simulink model "XYZCartesianRobot3DPrinting"  (R2024a)
settings: Solver=daessc  StartTime=0.0  StopTime=30  RelTol=1e-3  AbsTol=1e-3
PostLoadFcn:
  | run('XYZGantryRobotParameters.m')
  | run('LoadGantryRobot');
undefined symbols (not defined in the file): Controller, Floor, PrintBed, PrintHead, Trajectory, X, Y, Z
libraries: fl_lib x22, slpidlib x22, nesl_utility x15, sm_lib x10, sdl_lib x6, simulink x6, ee_lib x3
(part 1 of 3)
settings Model: Creator=abirdas  LastModifiedBy=abirdas
settings SolverCC: AutoScaleAbsTol=off
settings DataIOCC: SignalLoggingName=logsoutCartesianRobot3DPrinting
settings SimscapeCC: SimscapeLogType=all  SimscapeLogDataHistory=10000000

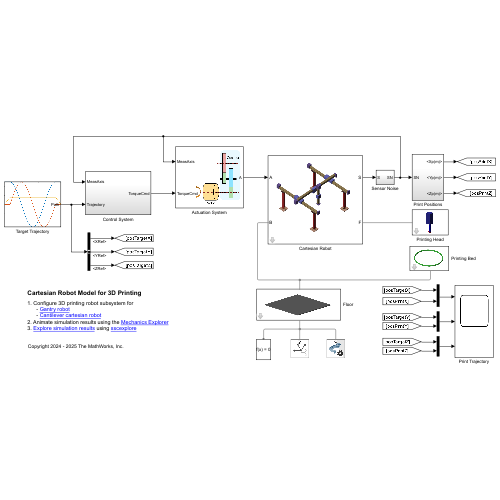
[thumbnail: Simulink's stored preview of the top-level diagram]
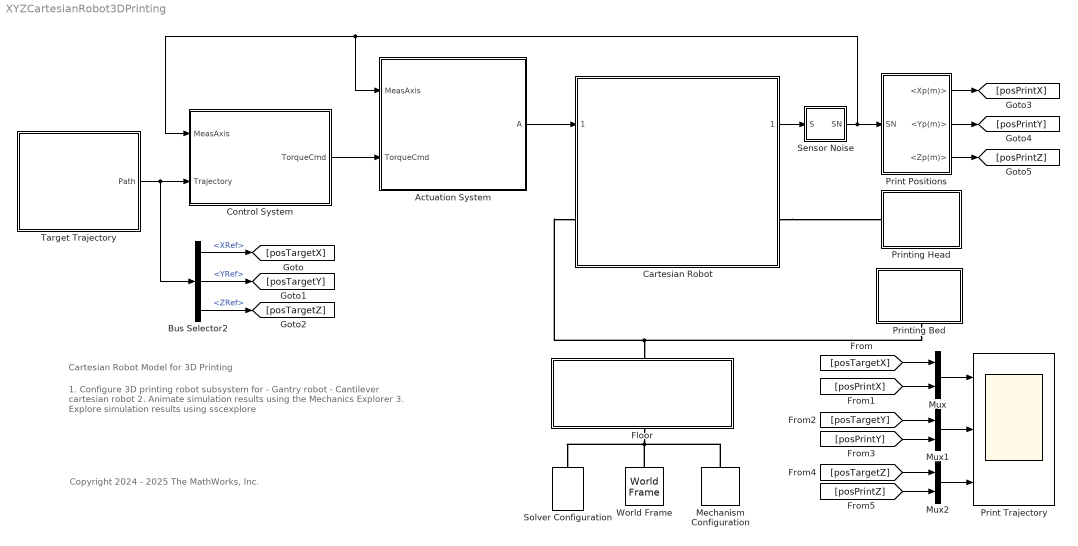
== system XYZCartesianRobot3DPrinting ==
  note: 1. Configure 3D printing robot subsystem for
      | - Gantry robot
      | - Cantilever cartesian robot
      | 2. Animate simulation results using the Mechanics Explorer
      | 3. Explore simulation results using sscexplore
  note: Cartesian Robot Model for 3D Printing
  note: Copyright 2024 - 2025 The MathWorks, Inc.
  Actuation System : Subsystem
      mask Display: image('ElectricalActuationSystem.png');
  Bus Selector2 : BusSelector  OutputSignals=XRef,YRef,ZRef
  Cartesian Robot : Subsystem  ReferencedSubsystem=GantryRobotSubsystem  DOF=3DOF  configAxis=XYZ  heightColumn=CartesianRobot.BaseFrame.heightColumn  widthColumn=CartesianRobot.BaseFrame.widthColumn  positionColumn1=CartesianRobot.BaseFrame.positionColumn1  positionColumn2=CartesianRobot.BaseFrame.positionColumn2  positionColumn3=CartesianRobot.BaseFrame.positionColumn3  positionColumn4=CartesianRobot.BaseFrame.positionColumn4  systemGuideX=Rail-block  strokeXMax=CartesianRobot.XAxis.strokeMax  widthGuideX=CartesianRobot.XAxis.widthRail  diaScrewX=0.05  widthXMount=0.3  typeInertiaGuideX=Calculate from Geometry  densityGuideX=CartesianRobot.XAxis.densityRail  massGuideX=0  COMGuideX=0  MOIGuideX=0  POIGuideX=0  typeInertiaCarriageX=Calculate from Geometry  densityCarriageX=CartesianRobot.XAxis.densityBlock  massCarriageX=0  COMCarriageX=0  MOICarriageX=0  POICarriageX=0  colorGuideX=[0.7 0.6 0.4]  colorCarriageX=[0.5 0.5 0.9]  systemGuideY=Rail-block  strokeYMax=CartesianRobot.YAxis.strokeMax  widthGuideY=CartesianRobot.YAxis.widthRail  diaScrewY=0.05  widthYMount=0.15  typeInertiaGuideY=Calculate from Geometry  densityGuideY=CartesianRobot.YAxis.densityRail  massGuideY=0  COMGuideY=0  MOIGuideY=0  POIGuideY=0  typeInertiaCarriageY=Calculate from Geometry  densityCarriageY=CartesianRobot.YAxis.densityBlock  massCarriageY=0  COMCarriageY=0  MOICarriageY=0  POICarriageY=0  colorGuideY=[0.7 0.6 0.4]  colorCarriageY=[0.5 0.5 0.9]  systemGuideZ=Rail-block  strokeZMax=CartesianRobot.ZAxis.strokeMax  widthGuideZ=CartesianRobot.ZAxis.widthRail  diaScrewZ=0.05  shiftZAxisDown=CartesianRobot.ZAxis.shiftZAxisDown  widthZMount=0.15  typeInertiaGuideZ=Calculate from Geometry  densityGuideZ=CartesianRobot.ZAxis.densityRail  massGuideZ=0  COMGuideZ=0  MOIGuideZ=0  POIGuideZ=0  typeInertiaCarriageZ=Calculate from Geometry  densityCarriageZ=CartesianRobot.ZAxis.densityBlock  massCarriageZ=0  COMCarriageZ=0  MOICarriageZ=0  POICarriageZ=0  colorGuideZ=[0.7 0.6 0.4]  colorCarriageZ=[0.5 0.5 0.9]
  Control System : Subsystem
  Floor : Subsystem  mask{floorDims=Floor.dimensions, floorPos=Floor.position}
      mask prompts: floorDims "Floor dimensions (m)"; floorPos "Floor position (m)"
      settings: PortSchema="{\"entries\":[{\"content\":{\"sides\":[{\"content\":{},\"type\":\"ConnectorPlacement.EquallySpacedRectSide\",\"uuid\":\"5b485af5-4f05-4248-a7f3-08377bf9cff2\"},{\"content\":{\"side\":\"RIGHT\"},\"type\":\"ConnectorPlacement.EquallySpacedRectSide\",\"uuid\":\"824380b3-967b-4422-aed9-09760effc9b4\"},{\"content\":{\"connectorIds\":[\"LConn1\"],\"side\":\"TOP\"},\"type\":\"ConnectorPlacement.EquallySpacedRectSide\",\"uuid\":\"4c7d634e-a270-49ee-a9b6-ce866eb97663\"},{\"content\":{\"connectorIds\":[\"RConn1\"],\"side\":\"BOTTOM\"},\"type\":\"ConnectorPlacement.EquallySpacedRectSide\",\"uuid\":\"d939dd98-fa2d-4b24-975e-597412481fcf\"}]},\"type\":\"ConnectorPlacement.EquallySpacedConnector\",\"uuid\":\"704e5fa1-0bef-4b5b-a1a4-570354550c26\"}],\"packageUris\":[\"http://schema.mathworks.com/mf0/Connector/R2020b\"],\"version\":\"1.0\"}"
      mask Display: image('Floor.png');
  Mechanism Configuration : sm_lib/Utilities/Mechanism Configuration  UniformGravity=Constant  GravityVector=[0 0 -9.80665]  GravityVectorUnits=m/s^2  LinearizationDelta=0.001  JointModeTransitionNonlinearIterations=2
  Mux : Mux  Inputs=2
  Mux1 : Mux  Inputs=2
  Mux2 : Mux  Inputs=2
  Print Positions : Subsystem
  Print Trajectory : Scope  NumInputPorts=3
  Printing Bed : Subsystem  mask{bedOffset=PrintBed.offsetFloor, bedRadius=PrintBed.radiusCircle, bedHeight=PrintBed.height, penThk=PrintHead.diaNozzleExit}
      mask prompts: bedOffset "Printing bed offset from floor (m)"; bedRadius "Printing bed radius (m)"; bedHeight "Printing bed height (m)"; penThk "Printing pen thickness (m)"
      mask init:
      | % Vertices of circular printing bed
      | v1 = [bedRadius + 0.5*penThk, 0];
      | v2 = [bedRadius + 0.5*penThk, bedHeight];
      | v3 = [bedRadius - 0.5*penThk, bedHeight];
      | v4 = [bedRadius - 0.5*penThk, 0];
      | sectionCircPrint = [v1; v2; v3; v4];
      settings: PortSchema="{\"entries\":[{\"content\":{\"sides\":[{\"content\":{},\"type\":\"ConnectorPlacement.EquallySpacedRectSide\",\"uuid\":\"5b485af5-4f05-4248-a7f3-08377bf9cff2\"},{\"content\":{\"side\":\"RIGHT\"},\"type\":\"ConnectorPlacement.EquallySpacedRectSide\",\"uuid\":\"824380b3-967b-4422-aed9-09760effc9b4\"},{\"content\":{\"side\":\"TOP\"},\"type\":\"ConnectorPlacement.EquallySpacedRectSide\",\"uuid\":\"4c7d634e-a270-49ee-a9b6-ce866eb97663\"},{\"content\":{\"connectorIds\":[\"RConn1\"],\"side\":\"BOTTOM\"},\"type\":\"ConnectorPlacement.EquallySpacedRectSide\",\"uuid\":\"d939dd98-fa2d-4b24-975e-597412481fcf\"}]},\"type\":\"ConnectorPlacement.EquallySpacedConnector\",\"uuid\":\"704e5fa1-0bef-4b5b-a1a4-570354550c26\"}],\"packageUris\":[\"http://schema.mathworks.com/mf0/Connector/R2020b\"],\"version\":\"1.0\"}"
      mask Display: image('AnnularPrintingBed.png');
  Printing Head : Subsystem  mask{dNozzle=PrintHead.diaNozzleExit}
      mask prompts: dNozzle "Nozzle exit diameter (m)"
      mask Display: image('PrintHead.png');
  Sensor Noise : Subsystem
  Solver Configuration : nesl_utility/Solver Configuration  PhysicalDomain=network_engine_domain  SubClassName=solver  LeftPortType=input  RightPortType=generic  Tones=[]  Harmonics=[]  SimulateNoise=off  Profile=off  UseLocalSampling=off  EnableSwitchedLinearOptims=on  FrequencyDomain=off  UseCCode=off  RelTol=0.001  AbsTol=0.001  MinStep=1e-09  ToWorkspace=off  RevertToSquareIcSolve=off  NumHomotopyIterations=100  PhasorMode=off  PhasorModeNumHarmonics=1  ConsistencySolver=NEWTON_XTOL_AFTER_FTOL  IndexReductionMethod=DerivativeReplacement  DoDC=off  ResidualTolerance=1e-09  ConsistencyTolSource=GLOBAL  ConsistencyAbsTol=0.001  ConsistencyRelTol=0.001  ConsistencyTolFactor=0.001  UseLocalSolver=off  LocalSolverChoice=NE_BACKWARD_EULER_ADVANCER  ResolveIndetEquations=on  FunctionEvalNumThread=1  LocalSolverSampleTime=0.001  DoFixedCost=off  MaxNonlinIter=3  MaxModeIter=2  ComputeImpulses=off  ImpulseIterations=2  LinearAlgebra=auto  LinearAlgebraNumThread=0  EquationFormulation=NE_TIME_EF  DelaysMemoryBudget=1024  AutomaticFiltering=on  FilteringTimeConstant=0.001  PartitionStorageMethod=AS_NEEDED  PartitionMemoryBudget=1024  PartitionMethod=ROBUST  MultibodyUseLocalSolver=off  MultibodyLocalSolverChoice=ODE1  MultibodyLocalSolverSampleTime=0.001
  Target Trajectory : Subsystem
      mask Display: image('MotionInputs.png');
  World Frame : sm_lib/Frames and Transforms/World Frame
  wires:
  Control System/1(TorqueCmd) -> Actuation System/2(TorqueCmd)
  Actuation System/1(A) -> Cartesian Robot/1
  Target Trajectory/1(Path) -> Control System/2(Trajectory), Bus Selector2/1
  Bus Selector2/3 -> [posTargetZ]  "<ZRef>"
  Bus Selector2/1 -> [posTargetX]  "<XRef>"
  Bus Selector2/2 -> [posTargetY]  "<YRef>"
  [posTargetY] -> Mux1/1
  Mux1/1 -> Print Trajectory/2
  Mux/1 -> Print Trajectory/1
  [posPrintZ] -> Mux2/2
  [posTargetZ] -> Mux2/1
  Mux2/1 -> Print Trajectory/3
  [posPrintX] -> Mux/2
  [posPrintY] -> Mux1/2
  [posTargetX] -> Mux/1
  Cartesian Robot/1 -> Sensor Noise/1(S)
  Sensor Noise/1(SN) -> Actuation System/1(MeasAxis), Control System/1(MeasAxis), Print Positions/1(SN)
  Print Positions/1(<Xp(m)>) -> [posPrintX]
  Print Positions/2(<Yp(m)>) -> [posPrintY]
  Print Positions/3(<Zp(m)>) -> [posPrintZ]
  connections:
  World Frame/RConn1 -- Solver Configuration/RConn1 -- Mechanism Configuration/RConn1 -- Floor/RConn1
  Printing Bed/RConn1 -- Cartesian Robot/LConn1 -- Floor/LConn1
  Cartesian Robot/RConn1 -- Printing Head/LConn1

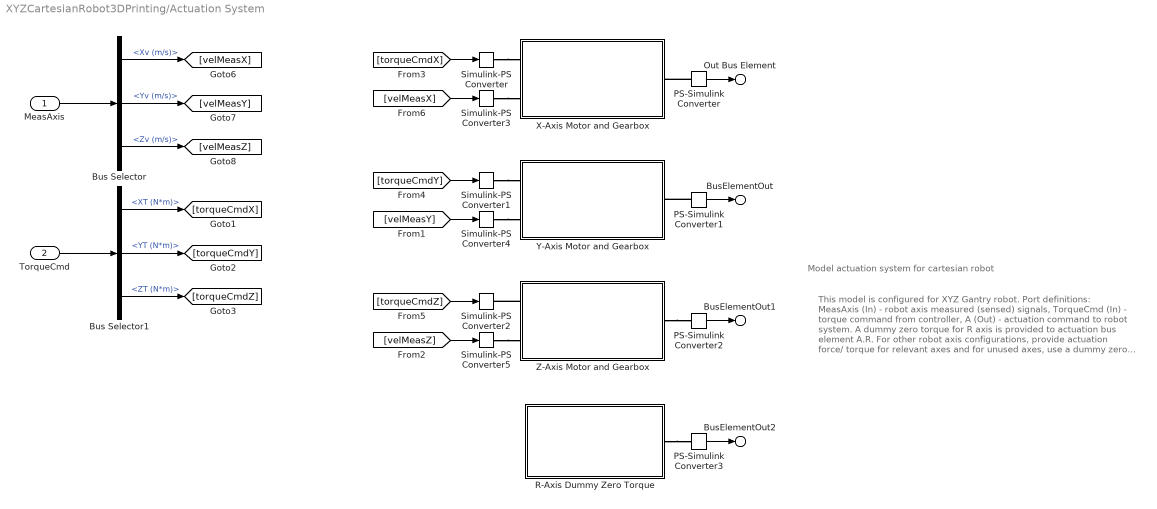
== system XYZCartesianRobot3DPrinting/Actuation System ==
  note: Model actuation system for cartesian robot
  note: This model is configured for XYZ Gantry robot.
      | Port definitions:
      | MeasAxis (In) - robot axis measured (sensed) signals,
      | TorqueCmd (In) - torque command from controller,
      | A (Out) - actuation command to robot system.
      |
      | A dummy zero torque for R axis is provided to actuation bus element A.R.
      | For other robot axis configurations, provide actuation force/ torque for relevant axes and for unused axes, use a dummy zero force/ torque.
  MeasAxis : Inport
  TorqueCmd : Inport  Port=2
  Bus Selector : BusSelector  OutputSignals=Xv (m/s),Yv (m/s),Zv (m/s)
  Bus Selector1 : BusSelector  OutputSignals=XT (N*m),YT (N*m),ZT (N*m)
  PS-Simulink Converter{,1..3} (4 alike) : nesl_utility/PS-Simulink Converter  PhysicalDomain=network_engine_domain  SubClassName=ps_output  LeftPortType=input  RightPortType=output  PseudoPeriodic=off  Frequencies=[]  VectorFormat=inherit  Unit=inherit  AffineConversion=off
  R-Axis Dummy Zero Torque : Subsystem
  Simulink-PS Converter : nesl_utility/Simulink-PS Converter  PhysicalDomain=network_engine_domain  SubClassName=ps_input  LeftPortType=input  RightPortType=output  PseudoPeriodic=off  Frequencies=[]  NoiseDistribution=none  NoiseParameters=[]  Unit=N*m  AffineConversion=off  FilteringAndDerivatives=provide  SimscapeFilterOrder=1  InputFilterTimeConstant=0.001  UdotUserProvided=0
  Simulink-PS Converter1 : nesl_utility/Simulink-PS Converter  PhysicalDomain=network_engine_domain  SubClassName=ps_input  LeftPortType=input  RightPortType=output  PseudoPeriodic=off  Frequencies=[]  NoiseDistribution=none  NoiseParameters=[]  Unit=N*m  AffineConversion=off  FilteringAndDerivatives=provide  SimscapeFilterOrder=1  InputFilterTimeConstant=0.001  UdotUserProvided=0
  Simulink-PS Converter2 : nesl_utility/Simulink-PS Converter  PhysicalDomain=network_engine_domain  SubClassName=ps_input  LeftPortType=input  RightPortType=output  PseudoPeriodic=off  Frequencies=[]  NoiseDistribution=none  NoiseParameters=[]  Unit=N*m  AffineConversion=off  FilteringAndDerivatives=provide  SimscapeFilterOrder=1  InputFilterTimeConstant=0.001  UdotUserProvided=0
  Simulink-PS Converter3 : nesl_utility/Simulink-PS Converter  PhysicalDomain=network_engine_domain  SubClassName=ps_input  LeftPortType=input  RightPortType=output  PseudoPeriodic=off  Frequencies=[]  NoiseDistribution=none  NoiseParameters=[]  Unit=m/s  AffineConversion=off  FilteringAndDerivatives=filter  SimscapeFilterOrder=1  InputFilterTimeConstant=0.001  UdotUserProvided=0
  Simulink-PS Converter4 : nesl_utility/Simulink-PS Converter  PhysicalDomain=network_engine_domain  SubClassName=ps_input  LeftPortType=input  RightPortType=output  PseudoPeriodic=off  Frequencies=[]  NoiseDistribution=none  NoiseParameters=[]  Unit=m/s  AffineConversion=off  FilteringAndDerivatives=filter  SimscapeFilterOrder=1  InputFilterTimeConstant=0.001  UdotUserProvided=0
  Simulink-PS Converter5 : nesl_utility/Simulink-PS Converter  PhysicalDomain=network_engine_domain  SubClassName=ps_input  LeftPortType=input  RightPortType=output  PseudoPeriodic=off  Frequencies=[]  NoiseDistribution=none  NoiseParameters=[]  Unit=m/s  AffineConversion=off  FilteringAndDerivatives=filter  SimscapeFilterOrder=1  InputFilterTimeConstant=0.001  UdotUserProvided=0
  X-Axis Motor and Gearbox : Subsystem
  Y-Axis Motor and Gearbox : Subsystem
  Z-Axis Motor and Gearbox : Subsystem
  Out Bus Element : Outport  PortName=A  Element=X
  BusElementOut : Outport  PortName=A  Element=Y
  BusElementOut1 : Outport  PortName=A  Element=Z
  BusElementOut2 : Outport  PortName=A  Element=R
  wires:
  MeasAxis/1 -> Bus Selector/1
  TorqueCmd/1 -> Bus Selector1/1
  Bus Selector1/1 -> [torqueCmdX]  "<XT (N*m)>"
  Bus Selector1/2 -> [torqueCmdY]  "<YT (N*m)>"
  Bus Selector1/3 -> [torqueCmdZ]  "<ZT (N*m)>"
  PS-Simulink Converter/1 -> Out Bus Element/1
  PS-Simulink Converter1/1 -> BusElementOut/1
  [velMeasX] -> Simulink-PS Converter3/1
  [velMeasY] -> Simulink-PS Converter4/1
  [velMeasZ] -> Simulink-PS Converter5/1
  [torqueCmdX] -> Simulink-PS Converter/1
  [torqueCmdY] -> Simulink-PS Converter1/1
  [torqueCmdZ] -> Simulink-PS Converter2/1
  PS-Simulink Converter3/1 -> BusElementOut2/1
  PS-Simulink Converter2/1 -> BusElementOut1/1
  Bus Selector/1 -> [velMeasX]  "<Xv (m/s)>"
  Bus Selector/2 -> [velMeasY]  "<Yv (m/s)>"
  Bus Selector/3 -> [velMeasZ]  "<Zv (m/s)>"
  connections:
  Z-Axis Motor and Gearbox/LConn1 -- Simulink-PS Converter2/RConn1
  Simulink-PS Converter/RConn1 -- X-Axis Motor and Gearbox/LConn1
  Simulink-PS Converter1/RConn1 -- Y-Axis Motor and Gearbox/LConn1
  PS-Simulink Converter/LConn1 -- X-Axis Motor and Gearbox/RConn1
  PS-Simulink Converter1/LConn1 -- Y-Axis Motor and Gearbox/RConn1
  Z-Axis Motor and Gearbox/RConn1 -- PS-Simulink Converter2/LConn1
  Simulink-PS Converter3/RConn1 -- X-Axis Motor and Gearbox/LConn2
  Simulink-PS Converter4/RConn1 -- Y-Axis Motor and Gearbox/LConn2
  Simulink-PS Converter5/RConn1 -- Z-Axis Motor and Gearbox/LConn2
  R-Axis Dummy Zero Torque/RConn1 -- PS-Simulink Converter3/LConn1

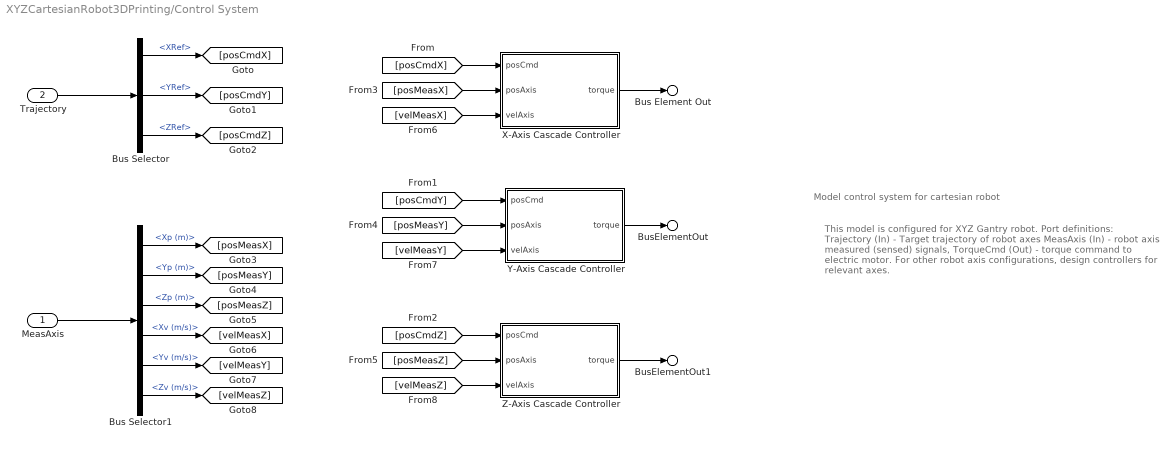
== system XYZCartesianRobot3DPrinting/Control System ==
  note: This model is configured for XYZ Gantry robot.
      | Port definitions:
      | Trajectory (In) - Target trajectory of robot axes
      | MeasAxis (In) - robot axis measured (sensed) signals,
      | TorqueCmd (Out) - torque command to electric motor.
      |
      | For other robot axis configurations, design controllers for relevant axes.
  note: Model control system for cartesian robot
  MeasAxis : Inport
  Trajectory : Inport  Port=2
  Bus Selector : BusSelector  OutputSignals=XRef,YRef,ZRef
  Bus Selector1 : BusSelector  OutputSignals=Xp (m),Yp (m),Zp (m),Xv (m/s),Yv (m/s),Zv (m/s)
  X-Axis Cascade Controller : Subsystem
  Y-Axis Cascade Controller : Subsystem
  Z-Axis Cascade Controller : Subsystem
  Bus Element Out : Outport  PortName=TorqueCmd  Element=XT (N*m)
  BusElementOut : Outport  PortName=TorqueCmd  Element=YT (N*m)
  BusElementOut1 : Outport  PortName=TorqueCmd  Element=ZT (N*m)
  wires:
  Trajectory/1 -> Bus Selector/1
  MeasAxis/1 -> Bus Selector1/1
  Bus Selector/1 -> [posCmdX]  "<XRef>"
  [posCmdX] -> X-Axis Cascade Controller/1(posCmd)
  Bus Selector/2 -> [posCmdY]  "<YRef>"
  Bus Selector/3 -> [posCmdZ]  "<ZRef>"
  [posCmdY] -> Y-Axis Cascade Controller/1(posCmd)
  [posCmdZ] -> Z-Axis Cascade Controller/1(posCmd)
  [posMeasX] -> X-Axis Cascade Controller/2(posAxis)
  [velMeasX] -> X-Axis Cascade Controller/3(velAxis)
  [posMeasY] -> Y-Axis Cascade Controller/2(posAxis)
  [velMeasY] -> Y-Axis Cascade Controller/3(velAxis)
  [posMeasZ] -> Z-Axis Cascade Controller/2(posAxis)
  [velMeasZ] -> Z-Axis Cascade Controller/3(velAxis)
  X-Axis Cascade Controller/1(torque) -> Bus Element Out/1
  Y-Axis Cascade Controller/1(torque) -> BusElementOut/1
  Z-Axis Cascade Controller/1(torque) -> BusElementOut1/1
  Bus Selector1/1 -> [posMeasX]  "<Xp (m)>"
  Bus Selector1/2 -> [posMeasY]  "<Yp (m)>"
  Bus Selector1/3 -> [posMeasZ]  "<Zp (m)>"
  Bus Selector1/4 -> [velMeasX]  "<Xv (m/s)>"
  Bus Selector1/5 -> [velMeasY]  "<Yv (m/s)>"
  Bus Selector1/6 -> [velMeasZ]  "<Zv (m/s)>"

== system XYZCartesianRobot3DPrinting/Floor ==
  Brick Solid : sm_lib/Body Elements/Brick Solid  BrickDimensions=floorDims  BrickDimensionsUnits=m  ExportEntireGeometry=off  InertiaType=CalculateFromGeometry  BasedOnType=Density  Density=1000  DensityUnits=kg/m^3  Mass=1  MassUnits=kg  CenterOfMass=[0 0 0]  CenterOfMassUnits=m  MomentsOfInertia=[1 1 1]  MomentsOfInertiaUnits=kg*m^2  ProductsOfInertia=[0 0 0]  ProductsOfInertiaUnits=kg*m^2  GraphicType=FromGeometry  MarkerShape=Sphere  MarkerSize=10  GraphicVisPropType=SimpleVisualProperties  GraphicDiffuseColor=[0.5 0.5 0.5]  GraphicOpacity=1  GraphicSpecularColor=[0.5 0.5 0.5 1.0]  GraphicAmbientColor=[0.15 0.15 0.15 1.0]  GraphicEmissiveColor=[0.0 0.0 0.0 1.0]  GraphicShininess=75  DoExposeReferenceFrame=off  SerializedFrames=<Frames><Frame><Id>Frame1</Id><Value><Name>F1</Name><Origin><Source>GeometricFeature</Source><FeatureName>-z surface</FeatureName></Origin><PrimaryAxis><DefinedDirection>+Z</DefinedDirection><Source>ReferenceFrame</Source><SourceDirection>+Z</SourceDirection><FeatureName></FeatureName></PrimaryAxis><SecondaryAxis><DefinedDirection>+X</DefinedDirection><Source>ReferenceFrame</Source><SourceDirection>+X</SourceDirection><FeatureName></FeatureName></SecondaryAxis></Value></Frame><Frame><Id>Frame2</Id><Value><Name>F2</Name><Origin><Source>GeometricFeature</Source><FeatureName>+z surface</FeatureName></Origin><PrimaryAxis><DefinedDirection>+Z</DefinedDirection><Source>ReferenceFrame</Source><SourceDirection>+Z</SourceDirection><FeatureName></FeatureName></PrimaryAxis><SecondaryAxis><DefinedDirection>+X</DefinedDirection><Source>ReferenceFrame</Source><SourceDirection>+X</SourceDirection><FeatureName></FeatureName></SecondaryAxis></Value></Frame></Frames>
  Rigid Transform : sm_lib/Frames and Transforms/Rigid Transform  RotationMethod=None  FollAlignAxisA=+X  BaseAlignAxisA=+Y  FollAlignAxisB=+Y  BaseAlignAxisB=+Z  RotationStandardAxis=+Z  RotationAngle=0  RotationAngleUnits=deg  RotationArbitraryAxis=[0 0 1]  RotationSequenceAxes=FollowerAxes  RotationSequence=XYX  RotationSequenceAngles=[0 0 0]  RotationSequenceAnglesUnits=deg  RotationMatrix=[1 0 0;0 1 0;0 0 1]  Quaternion=[1 0 0 0]  TranslationMethod=Cartesian  TranslationCartesianOffset=floorPos  TranslationCartesianOffsetUnits=m  TranslationStandardAxis=+Z  TranslationStandardOffset=0  TranslationStandardOffsetUnits=m  TranslationROffset=0  TranslationROffsetUnits=m  TranslationThetaOffset=0  TranslationThetaOffsetUnits=deg  TranslationZOffset=0  TranslationZOffsetUnits=m
  Rigid Transform1 : sm_lib/Frames and Transforms/Rigid Transform  RotationMethod=None  FollAlignAxisA=+X  BaseAlignAxisA=+Y  FollAlignAxisB=+Y  BaseAlignAxisB=+Z  RotationStandardAxis=+Z  RotationAngle=0  RotationAngleUnits=deg  RotationArbitraryAxis=[0 0 1]  RotationSequenceAxes=FollowerAxes  RotationSequence=XYX  RotationSequenceAngles=[0 0 0]  RotationSequenceAnglesUnits=deg  RotationMatrix=[1 0 0;0 1 0;0 0 1]  Quaternion=[1 0 0 0]  TranslationMethod=Cartesian  TranslationCartesianOffset=-floorPos  TranslationCartesianOffsetUnits=m  TranslationStandardAxis=+Z  TranslationStandardOffset=0  TranslationStandardOffsetUnits=m  TranslationROffset=0  TranslationROffsetUnits=m  TranslationThetaOffset=0  TranslationThetaOffsetUnits=deg  TranslationZOffset=0  TranslationZOffsetUnits=m
  F : PMIOPort  Side=Left
  B : PMIOPort  Port=2  Side=Right
  connections:
  F/RConn1 -- Rigid Transform1/RConn1
  Rigid Transform/RConn1 -- Brick Solid/LConn1
  B/RConn1 -- Rigid Transform/LConn1
  Rigid Transform1/LConn1 -- Brick Solid/RConn1

== system XYZCartesianRobot3DPrinting/Print Positions ==
  SN : Inport
  Bus Selector3 : BusSelector  OutputSignals=Xp (m),Yp (m),Zp (m)
  Constant1 : Constant  Value=PrintHead.offsetX %Trajectory.radiusCircle
  Sum1 : Sum  Inputs=|++
  <Xp(m)> : Outport
  <Yp(m)> : Outport  Port=2
  <Zp(m)> : Outport  Port=3
  wires:
  SN/1 -> Bus Selector3/1
  Bus Selector3/3 -> <Zp(m)>/1  "<Zp (m)>"
  Bus Selector3/2 -> <Yp(m)>/1  "<Yp (m)>"
  Sum1/1 -> <Xp(m)>/1  "<Xp (m)>"
  Bus Selector3/1 -> Sum1/1  "<Xp (m)>"
  Constant1/1 -> Sum1/2

== system XYZCartesianRobot3DPrinting/Printing Bed ==
  Revolved Solid : sm_lib/Body Elements/Revolved Solid  RevolutionCrossSection=sectionCircPrint  RevolutionCrossSectionUnits=m  RevolutionExtent=Full  RevolutionAngle=180  RevolutionAngleUnits=deg  ExportConvexHullGeometry=off  InertiaType=CalculateFromGeometry  BasedOnType=Density  Density=1000  DensityUnits=kg/m^3  Mass=1  MassUnits=kg  CenterOfMass=[0 0 0]  CenterOfMassUnits=m  MomentsOfInertia=[1 1 1]  MomentsOfInertiaUnits=kg*m^2  ProductsOfInertia=[0 0 0]  ProductsOfInertiaUnits=kg*m^2  GraphicType=FromGeometry  MarkerShape=Sphere  MarkerSize=10  GraphicVisPropType=SimpleVisualProperties  GraphicDiffuseColor=[0.3 0.9 0.3]  GraphicOpacity=1  GraphicSpecularColor=[0.5 0.5 0.5 1.0]  GraphicAmbientColor=[0.15 0.15 0.15 1.0]  GraphicEmissiveColor=[0.0 0.0 0.0 1.0]  GraphicShininess=75  DoExposeReferenceFrame=off  SerializedFrames=<Frames><Frame><Id>Frame1</Id><Value><Name>F1</Name><Origin><Source>GeometricFeature</Source><FeatureName>side surface 4</FeatureName></Origin><PrimaryAxis><DefinedDirection>+Z</DefinedDirection><Source>ReferenceFrame</Source><SourceDirection>+Z</SourceDirection><FeatureName></FeatureName></PrimaryAxis><SecondaryAxis><DefinedDirection>+X</DefinedDirection><Source>ReferenceFrame</Source><SourceDirection>+X</SourceDirection><FeatureName></FeatureName></SecondaryAxis></Value></Frame></Frames>
  Rigid Transform : sm_lib/Frames and Transforms/Rigid Transform  RotationMethod=None  FollAlignAxisA=+X  BaseAlignAxisA=+Y  FollAlignAxisB=+Y  BaseAlignAxisB=+Z  RotationStandardAxis=+Z  RotationAngle=0  RotationAngleUnits=deg  RotationArbitraryAxis=[0 0 1]  RotationSequenceAxes=FollowerAxes  RotationSequence=XYX  RotationSequenceAngles=[0 0 0]  RotationSequenceAnglesUnits=deg  RotationMatrix=[1 0 0;0 1 0;0 0 1]  Quaternion=[1 0 0 0]  TranslationMethod=Cartesian  TranslationCartesianOffset=bedOffset  TranslationCartesianOffsetUnits=m  TranslationStandardAxis=+Z  TranslationStandardOffset=0  TranslationStandardOffsetUnits=m  TranslationROffset=0  TranslationROffsetUnits=m  TranslationThetaOffset=0  TranslationThetaOffsetUnits=deg  TranslationZOffset=0  TranslationZOffsetUnits=m
  B : PMIOPort  Side=Right
  connections:
  Revolved Solid/LConn1 -- Rigid Transform/RConn1
  B/RConn1 -- Rigid Transform/LConn1

== system XYZCartesianRobot3DPrinting/Printing Head ==
  Body : sm_lib/Body Elements/Brick Solid  BrickDimensions=[5*dNozzle 5*dNozzle 20*dNozzle]  BrickDimensionsUnits=m  ExportEntireGeometry=off  InertiaType=CalculateFromGeometry  BasedOnType=Density  Density=1000  DensityUnits=kg/m^3  Mass=1  MassUnits=kg  CenterOfMass=[0 0 0]  CenterOfMassUnits=m  MomentsOfInertia=[1 1 1]  MomentsOfInertiaUnits=kg*m^2  ProductsOfInertia=[0 0 0]  ProductsOfInertiaUnits=kg*m^2  GraphicType=FromGeometry  MarkerShape=Sphere  MarkerSize=10  GraphicVisPropType=SimpleVisualProperties  GraphicDiffuseColor=[0.2 0.2 0.7]  GraphicOpacity=1  GraphicSpecularColor=[0.5 0.5 0.5 1.0]  GraphicAmbientColor=[0.15 0.15 0.15 1.0]  GraphicEmissiveColor=[0.0 0.0 0.0 1.0]  GraphicShininess=75  DoExposeReferenceFrame=off  SerializedFrames=<Frames><Frame><Id>Frame1</Id><Value><Name>F1</Name><Origin><Source>GeometricFeature</Source><FeatureName>-x surface</FeatureName></Origin><PrimaryAxis><DefinedDirection>+Z</DefinedDirection><Source>ReferenceFrame</Source><SourceDirection>+Z</SourceDirection><FeatureName></FeatureName></PrimaryAxis><SecondaryAxis><DefinedDirection>+X</DefinedDirection><Source>ReferenceFrame</Source><SourceDirection>+X</SourceDirection><FeatureName></FeatureName></SecondaryAxis></Value></Frame><Frame><Id>Frame2</Id><Value><Name>F2</Name><Origin><Source>GeometricFeature</Source><FeatureName>-z surface</FeatureName></Origin><PrimaryAxis><DefinedDirection>+Z</DefinedDirection><Source>ReferenceFrame</Source><SourceDirection>+Z</SourceDirection><FeatureName></FeatureName></PrimaryAxis><SecondaryAxis><DefinedDirection>+X</DefinedDirection><Source>ReferenceFrame</Source><SourceDirection>+X</SourceDirection><FeatureName></FeatureName></SecondaryAxis></Value></Frame></Frames>
  Nozzle : sm_lib/Body Elements/Revolved Solid  RevolutionCrossSection=[0.5*dNozzle 0; 1.5*dNozzle 3*dNozzle; 0 3*dNozzle; 0 0]  RevolutionCrossSectionUnits=m  RevolutionExtent=Full  RevolutionAngle=180  RevolutionAngleUnits=deg  ExportConvexHullGeometry=off  InertiaType=CalculateFromGeometry  BasedOnType=Density  Density=1000  DensityUnits=kg/m^3  Mass=1  MassUnits=kg  CenterOfMass=[0 0 0]  CenterOfMassUnits=m  MomentsOfInertia=[1 1 1]  MomentsOfInertiaUnits=kg*m^2  ProductsOfInertia=[0 0 0]  ProductsOfInertiaUnits=kg*m^2  GraphicType=FromGeometry  MarkerShape=Sphere  MarkerSize=10  GraphicVisPropType=SimpleVisualProperties  GraphicDiffuseColor=[0.9 0.1 0.1]  GraphicOpacity=1  GraphicSpecularColor=[0.5 0.5 0.5 1.0]  GraphicAmbientColor=[0.15 0.15 0.15 1.0]  GraphicEmissiveColor=[0.0 0.0 0.0 1.0]  GraphicShininess=75  DoExposeReferenceFrame=off  SerializedFrames=<Frames><Frame><Id>Frame1</Id><Value><Name>F1</Name><Origin><Source>GeometricFeature</Source><FeatureName>side surface 2</FeatureName></Origin><PrimaryAxis><DefinedDirection>+Z</DefinedDirection><Source>ReferenceFrame</Source><SourceDirection>+Z</SourceDirection><FeatureName></FeatureName></PrimaryAxis><SecondaryAxis><DefinedDirection>+X</DefinedDirection><Source>ReferenceFrame</Source><SourceDirection>+X</SourceDirection><FeatureName></FeatureName></SecondaryAxis></Value></Frame></Frames>
  Pipe : sm_lib/Body Elements/Cylindrical Solid  CylinderRadius=dNozzle  CylinderRadiusUnits=m  CylinderLength=15*dNozzle  CylinderLengthUnits=m  ExportEntireGeometry=off  InertiaType=CalculateFromGeometry  BasedOnType=Density  Density=1000  DensityUnits=kg/m^3  Mass=1  MassUnits=kg  CenterOfMass=[0 0 0]  CenterOfMassUnits=m  MomentsOfInertia=[1 1 1]  MomentsOfInertiaUnits=kg*m^2  ProductsOfInertia=[0 0 0]  ProductsOfInertiaUnits=kg*m^2  GraphicType=FromGeometry  MarkerShape=Sphere  MarkerSize=10  GraphicVisPropType=SimpleVisualProperties  GraphicDiffuseColor=[0 0 1]  GraphicOpacity=1  GraphicSpecularColor=[0.5 0.5 0.5 1.0]  GraphicAmbientColor=[0.15 0.15 0.15 1.0]  GraphicEmissiveColor=[0.0 0.0 0.0 1.0]  GraphicShininess=75  DoExposeReferenceFrame=off  SerializedFrames=<Frames><Frame><Id>Frame1</Id><Value><Name>F1</Name><Origin><Source>GeometricFeature</Source><FeatureName>top surface</FeatureName></Origin><PrimaryAxis><DefinedDirection>+Z</DefinedDirection><Source>ReferenceFrame</Source><SourceDirection>+Z</SourceDirection><FeatureName></FeatureName></PrimaryAxis><SecondaryAxis><DefinedDirection>+X</DefinedDirection><Source>ReferenceFrame</Source><SourceDirection>+X</SourceDirection><FeatureName></FeatureName></SecondaryAxis></Value></Frame><Frame><Id>Frame2</Id><Value><Name>F2</Name><Origin><Source>GeometricFeature</Source><FeatureName>bottom surface</FeatureName></Origin><PrimaryAxis><DefinedDirection>+Z</DefinedDirection><Source>ReferenceFrame</Source><SourceDirection>+Z</SourceDirection><FeatureName></FeatureName></PrimaryAxis><SecondaryAxis><DefinedDirection>+X</DefinedDirection><Source>ReferenceFrame</Source><SourceDirection>+X</SourceDirection><FeatureName></FeatureName></SecondaryAxis></Value></Frame></Frames>
  B : PMIOPort  Side=Left
  connections:
  Pipe/LConn1 -- Body/RConn1
  Nozzle/LConn1 -- Pipe/RConn1
  B/RConn1 -- Body/LConn1

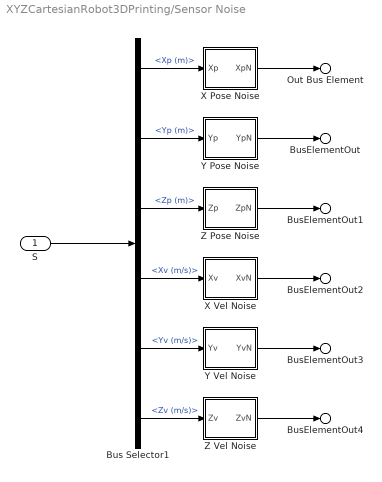
== system XYZCartesianRobot3DPrinting/Sensor Noise ==
  S : Inport
  Bus Selector1 : BusSelector  OutputSignals=XS.Xp (m),YS.Yp (m),ZS.Zp (m),XS.Xv (m/s),YS.Yv (m/s),ZS.Zv (m/s)
  X Pose Noise : Subsystem
  X Vel Noise : Subsystem
  Y Pose Noise : Subsystem
  Y Vel Noise : Subsystem
  Z Pose Noise : Subsystem
  Z Vel Noise : Subsystem
  Out Bus Element : Outport  PortName=SN  Element=Xp (m)
  BusElementOut : Outport  PortName=SN  Element=Yp (m)
  BusElementOut1 : Outport  PortName=SN  Element=Zp (m)
  BusElementOut2 : Outport  PortName=SN  Element=Xv (m/s)
  BusElementOut3 : Outport  PortName=SN  Element=Yv (m/s)
  BusElementOut4 : Outport  PortName=SN  Element=Zv (m/s)
  wires:
  S/1 -> Bus Selector1/1
  X Pose Noise/1(XpN) -> Out Bus Element/1
  Y Pose Noise/1(YpN) -> BusElementOut/1
  Z Pose Noise/1(ZpN) -> BusElementOut1/1
  X Vel Noise/1(XvN) -> BusElementOut2/1
  Y Vel Noise/1(YvN) -> BusElementOut3/1
  Z Vel Noise/1(ZvN) -> BusElementOut4/1
  Bus Selector1/1 -> X Pose Noise/1(Xp)  "<Xp (m)>"
  Bus Selector1/2 -> Y Pose Noise/1(Yp)  "<Yp (m)>"
  Bus Selector1/3 -> Z Pose Noise/1(Zp)  "<Zp (m)>"
  Bus Selector1/4 -> X Vel Noise/1(Xv)  "<Xv (m/s)>"
  Bus Selector1/5 -> Y Vel Noise/1(Yv)  "<Yv (m/s)>"
  Bus Selector1/6 -> Z Vel Noise/1(Zv)  "<Zv (m/s)>"

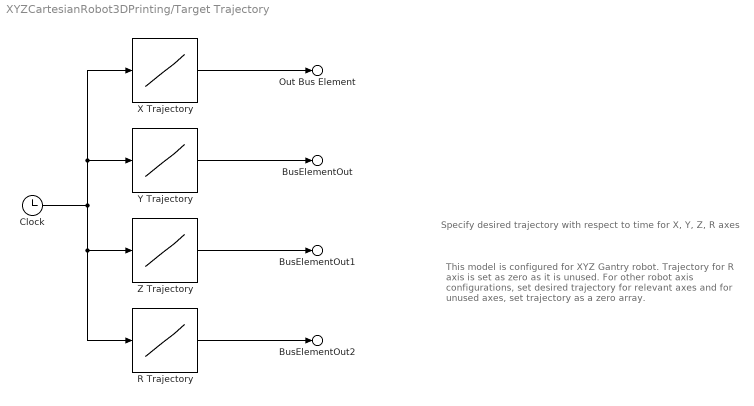
== system XYZCartesianRobot3DPrinting/Target Trajectory ==
  note: Specify desired trajectory with respect to time
      | for X, Y, Z, R axes
  note: This model is configured for XYZ Gantry robot.
      | Trajectory for R axis is set as zero as it is unused.
      | For other robot axis configurations, set desired trajectory for relevant axes and for unused axes, set trajectory as a zero array.
  Clock : Clock
  R Trajectory : Lookup_n-D  NumberOfTableDimensions=1  BreakpointsForDimension1=Trajectory.time  Table=Trajectory.pathR  InternalRulePriority=Speed  RndMeth=Simplest
  X Trajectory : Lookup_n-D  NumberOfTableDimensions=1  BreakpointsForDimension1=Trajectory.time  Table=Trajectory.pathX  InternalRulePriority=Speed  RndMeth=Simplest
  Y Trajectory : Lookup_n-D  NumberOfTableDimensions=1  BreakpointsForDimension1=Trajectory.time  Table=Trajectory.pathY  InternalRulePriority=Speed  RndMeth=Simplest
  Z Trajectory : Lookup_n-D  NumberOfTableDimensions=1  BreakpointsForDimension1=Trajectory.time  Table=Trajectory.pathZ  InternalRulePriority=Speed  RndMeth=Simplest
  Out Bus Element : Outport  PortName=Path  Element=XRef
  BusElementOut : Outport  PortName=Path  Element=YRef
  BusElementOut1 : Outport  PortName=Path  Element=ZRef
  BusElementOut2 : Outport  PortName=Path  Element=RRef
  wires:
  Clock/1 -> X Trajectory/1, Y Trajectory/1, R Trajectory/1, Z Trajectory/1
  X Trajectory/1 -> Out Bus Element/1
  Z Trajectory/1 -> BusElementOut1/1
  Y Trajectory/1 -> BusElementOut/1
  R Trajectory/1 -> BusElementOut2/1

== system XYZCartesianRobot3DPrinting/Actuation System/R-Axis Dummy Zero Torque ==
  PS Ramp : fl_lib/Physical Signals/Sources/PS Ramp  slope=0 N*m/s  start_time=0 s  initial_output=0 N*m
  Solver Configuration : nesl_utility/Solver Configuration  PhysicalDomain=network_engine_domain  SubClassName=solver  LeftPortType=input  RightPortType=generic  Tones=[]  Harmonics=[]  SimulateNoise=off  Profile=off  UseLocalSampling=off  EnableSwitchedLinearOptims=on  FrequencyDomain=off  UseCCode=off  RelTol=0.001  AbsTol=0.001  MinStep=1e-09  ToWorkspace=off  RevertToSquareIcSolve=off  NumHomotopyIterations=100  PhasorMode=off  PhasorModeNumHarmonics=1  ConsistencySolver=NEWTON_XTOL_AFTER_FTOL  IndexReductionMethod=DerivativeReplacement  DoDC=off  ResidualTolerance=1e-09  ConsistencyTolSource=GLOBAL  ConsistencyAbsTol=0.001  ConsistencyRelTol=0.001  ConsistencyTolFactor=0.001  UseLocalSolver=off  LocalSolverChoice=NE_BACKWARD_EULER_ADVANCER  ResolveIndetEquations=on  FunctionEvalNumThread=1  LocalSolverSampleTime=0.001  DoFixedCost=off  MaxNonlinIter=3  MaxModeIter=2  ComputeImpulses=off  ImpulseIterations=2  LinearAlgebra=auto  LinearAlgebraNumThread=0  EquationFormulation=NE_TIME_EF  DelaysMemoryBudget=1024  AutomaticFiltering=on  FilteringTimeConstant=0.001  PartitionStorageMethod=AS_NEEDED  PartitionMemoryBudget=1024  PartitionMethod=ROBUST  MultibodyUseLocalSolver=off  MultibodyLocalSolverChoice=ODE1  MultibodyLocalSolverSampleTime=0.001
  Torque : PMIOPort  Side=Right
  connections:
  PS Ramp/RConn1 -- Solver Configuration/RConn1 -- Torque/RConn1

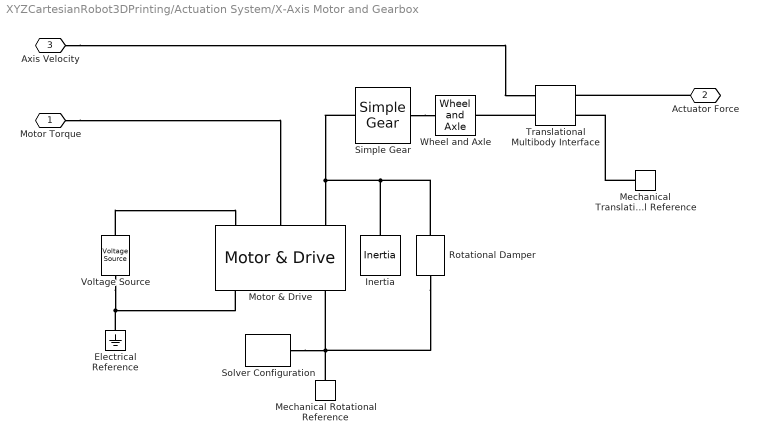
== system XYZCartesianRobot3DPrinting/Actuation System/X-Axis Motor and Gearbox ==
  Electrical Reference : fl_lib/Electrical/Electrical Elements/Electrical Reference
  Inertia : fl_lib/Mechanical/Rotational Elements/Inertia  inertia=0.0001 kg*m^2  num_ports=foundation.enum.numPorts2.one  w_specify=on  w_priority=Low  w=0 rad/s  w_nominal_specify=off  w_nominal_value=1  w_nominal_unit=rad/s  t_specify=off  t_priority=None  t=0 N*m  t_nominal_specify=off  t_nominal_value=1  t_nominal_unit=N*m
  Mechanical Rotational Reference : fl_lib/Mechanical/Rotational Elements/Mechanical Rotational Reference
  Mechanical Translational Reference : fl_lib/Mechanical/Translational Elements/Mechanical Translational Reference
  Motor & Drive : sdl_lib/Engines & Motors/Motor & Drive  torque_max=Actuation.XAxis.maxTorque N*m  power_max=Actuation.XAxis.maxPower kW  Tc=0.1 s  eff=100  w_eff=2000 rpm  T_eff=7 N*m  thermal_port=simscape.enum.thermaleffects.omit  thermal_mass=100 J/K  temperature_specify=off  temperature_priority=High  temperature=300 K  temperature_nominal_specify=off  temperature_nominal_value=1  temperature_nominal_unit=K
      settings: InternalSimscapePortConfiguration="{\"Bottom\":[],\"Left\":[{\"id\":\"Vp\",\"label\":\"+\",\"type\":\"foundation.electrical.electrical\"},{\"id\":\"Tr\",\"label\":\"Tr\",\"type\":\"input\"},{\"id\":\"R\",\"label\":\"R\",\"type\":\"foundation.mechanical.rotational.rotational\"}],\"Right\":[{\"id\":\"Vm\",\"label\":\"-\",\"type\":\"foundation.electrical.electrical\"},{\"id\":\"Omega\",\"label\":\"w\",\"type\":\"output\"},{\"id\":\"C\",\"label\":\"C\",\"type\":\"foundation.mechanical.rotational.rotational\"}],\"Top\":[]}"
  Rotational Damper : fl_lib/Mechanical/Rotational Elements/Rotational Damper  D=0.01 %0.0001 %0.1 N*m*s/rad  w_specify=off  w_priority=None  w=0 rad/s  w_nominal_specify=off  w_nominal_value=1  w_nominal_unit=rad/s  t_specify=off  t_priority=None  t=0 N*m  t_nominal_specify=off  t_nominal_value=1  t_nominal_unit=N*m
  Simple Gear : sdl_lib/Gears/Simple Gear  ratio=5  rotation_direction=sdl.enum.shaftOutputDirection.same  enable_faults=simscape.enum.onoff.off  efficiency_fault=0.05  fault_angles=pi / 12 rad  friction_model=sdl.enum.gear_efficiencies_load.off  T_noload=0.1 N*m  T_nom=5 N*m  efficiency_nom=0.8  efficiency=0.8  temperature_TLU=[280, 300, 320] K  load_TLU=[1, 5, 10] N*m  efficiency_TLU=[.95, .9, .85]  efficiency_TLU2=[.85, .8, .75; .95, .9, .85; .85, .8, .7]  w_thr=0.01 rad/s  pwr_thr=0.001 W  enable_backlash=false  hardstop_model=simscape.enum.hardstop.smooth  backlash_distance=1e-3 mm  r_base=0.1 m  transition=1e-4 mm  backlash_stiffness=1e6 N/m  backlash_damping=1e3 N*s/m  coeff_rest=0.7  v_tol=0.001 m/s  f_tol=0.001 N  mu_visc=[0, 0] N*m*s/rad  thermal_mass=50 J/K  temperature_specify=off  temperature_priority=High  temperature=300 K  temperature_nominal_specify=off  temperature_nominal_value=1  temperature_nominal_unit=K  x_backlash_specify=off  x_backlash_priority=None  x_backlash=0 mm  x_backlash_nominal_specify=off  x_backlash_nominal_value=1  x_backlash_nominal_unit=mm  f_hardstop_specify=off  f_hardstop_priority=None  f_hardstop=0 N  f_hardstop_nominal_specify=off  f_hardstop_nominal_value=1  f_hardstop_nominal_unit=N  v_backlash_specify=off  v_backlash_priority=None  v_backlash=0 m/s  v_backlash_nominal_specify=off  v_backlash_nominal_value=1  v_backlash_nominal_unit=m/s
  Solver Configuration : nesl_utility/Solver Configuration  PhysicalDomain=network_engine_domain  SubClassName=solver  LeftPortType=input  RightPortType=generic  Tones=[]  Harmonics=[]  SimulateNoise=off  Profile=off  UseLocalSampling=off  EnableSwitchedLinearOptims=on  FrequencyDomain=off  UseCCode=off  RelTol=0.001  AbsTol=0.001  MinStep=1e-09  ToWorkspace=off  RevertToSquareIcSolve=off  NumHomotopyIterations=100  PhasorMode=off  PhasorModeNumHarmonics=1  ConsistencySolver=NEWTON_XTOL_AFTER_FTOL  IndexReductionMethod=DerivativeReplacement  DoDC=off  ResidualTolerance=1e-09  ConsistencyTolSource=GLOBAL  ConsistencyAbsTol=0.001  ConsistencyRelTol=0.001  ConsistencyTolFactor=0.001  UseLocalSolver=off  LocalSolverChoice=NE_BACKWARD_EULER_ADVANCER  ResolveIndetEquations=on  FunctionEvalNumThread=1  LocalSolverSampleTime=0.001  DoFixedCost=off  MaxNonlinIter=3  MaxModeIter=2  ComputeImpulses=off  ImpulseIterations=2  LinearAlgebra=auto  LinearAlgebraNumThread=0  EquationFormulation=NE_TIME_EF  DelaysMemoryBudget=1024  AutomaticFiltering=on  FilteringTimeConstant=0.001  PartitionStorageMethod=AS_NEEDED  PartitionMemoryBudget=1024  PartitionMethod=ROBUST  MultibodyUseLocalSolver=off  MultibodyLocalSolverChoice=ODE1  MultibodyLocalSolverSampleTime=0.001
  Translational Multibody Interface : fl_lib/Mechanical/Multibody Interfaces/Translational Multibody Interface
  Voltage Source : ee_lib/Sources/Voltage Source  dc_voltage=48 %100 V  ac_voltage=0 V  ac_shift=0 rad  ac_frequency=60 Hz  noise_mode=ee.enum.sources.noise.Disabled  PSD=0 V^2/Hz  sample_time=1e-3 s  repeatability=ee.enum.sources.repeatability.NotRepeatable  user_seed=0  auto_seed=3499211588  i_specify=off  i_priority=None  i=0 A  i_nominal_specify=off  i_nominal_value=1  i_nominal_unit=A  v_specify=off  v_priority=None  v=0 V  v_nominal_specify=off  v_nominal_value=1  v_nominal_unit=V
  Wheel and Axle : fl_lib/Mechanical/Mechanisms/Wheel and Axle  R=0.071 m  or=1  t_specify=off  t_priority=None  t=0 N*m  t_nominal_specify=off  t_nominal_value=1  t_nominal_unit=N*m  f_specify=off  f_priority=None  f=0 N  f_nominal_specify=off  f_nominal_value=1  f_nominal_unit=N
  Motor Torque : PMIOPort  Side=Left
  Actuator Force : PMIOPort  Port=2  Side=Right
  Axis Velocity : PMIOPort  Port=3  Side=Left
  connections:
  Simple Gear/RConn1 -- Wheel and Axle/LConn1
  Inertia/LConn1 -- Simple Gear/LConn1 -- Motor & Drive/LConn3 -- Rotational Damper/LConn1
  Voltage Source/LConn1 -- Motor & Drive/LConn1
  Voltage Source/RConn1 -- Electrical Reference/LConn1 -- Motor & Drive/RConn1
  Mechanical Rotational Reference/LConn1 -- Solver Configuration/RConn1 -- Rotational Damper/RConn1 -- Motor & Drive/RConn3
  Motor Torque/RConn1 -- Motor & Drive/LConn2
  Translational Multibody Interface/RConn2 -- Wheel and Axle/RConn1
  Actuator Force/RConn1 -- Translational Multibody Interface/LConn1
  Mechanical Translational Reference/LConn1 -- Translational Multibody Interface/LConn2
  Axis Velocity/RConn1 -- Translational Multibody Interface/RConn1

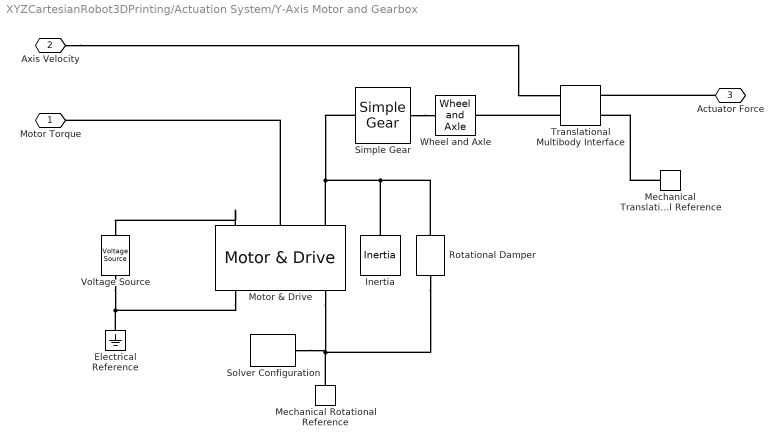
== system XYZCartesianRobot3DPrinting/Actuation System/Y-Axis Motor and Gearbox ==
  Electrical Reference : fl_lib/Electrical/Electrical Elements/Electrical Reference
  Inertia : fl_lib/Mechanical/Rotational Elements/Inertia  inertia=1e-5 %0.0001 kg*m^2  num_ports=foundation.enum.numPorts2.one  w_specify=on  w_priority=Low  w=0 rad/s  w_nominal_specify=off  w_nominal_value=1  w_nominal_unit=rad/s  t_specify=off  t_priority=None  t=0 N*m  t_nominal_specify=off  t_nominal_value=1  t_nominal_unit=N*m
  Mechanical Rotational Reference : fl_lib/Mechanical/Rotational Elements/Mechanical Rotational Reference
  Mechanical Translational Reference : fl_lib/Mechanical/Translational Elements/Mechanical Translational Reference
  Motor & Drive : sdl_lib/Engines & Motors/Motor & Drive  torque_max=Actuation.YAxis.maxTorque N*m  power_max=Actuation.YAxis.maxPower kW  Tc=0.1 s  eff=100  w_eff=2000 rpm  T_eff=7 N*m  thermal_port=simscape.enum.thermaleffects.omit  thermal_mass=100 J/K  temperature_specify=off  temperature_priority=High  temperature=300 K  temperature_nominal_specify=off  temperature_nominal_value=1  temperature_nominal_unit=K
      settings: InternalSimscapePortConfiguration="{\"Bottom\":[],\"Left\":[{\"id\":\"Vp\",\"label\":\"+\",\"type\":\"foundation.electrical.electrical\"},{\"id\":\"Tr\",\"label\":\"Tr\",\"type\":\"input\"},{\"id\":\"R\",\"label\":\"R\",\"type\":\"foundation.mechanical.rotational.rotational\"}],\"Right\":[{\"id\":\"Vm\",\"label\":\"-\",\"type\":\"foundation.electrical.electrical\"},{\"id\":\"Omega\",\"label\":\"w\",\"type\":\"output\"},{\"id\":\"C\",\"label\":\"C\",\"type\":\"foundation.mechanical.rotational.rotational\"}],\"Top\":[]}"
  Rotational Damper : fl_lib/Mechanical/Rotational Elements/Rotational Damper  D=0.01 %0.0001 %0.1 N*m*s/rad  w_specify=off  w_priority=None  w=0 rad/s  w_nominal_specify=off  w_nominal_value=1  w_nominal_unit=rad/s  t_specify=off  t_priority=None  t=0 N*m  t_nominal_specify=off  t_nominal_value=1  t_nominal_unit=N*m
  Simple Gear : sdl_lib/Gears/Simple Gear  ratio=5  rotation_direction=sdl.enum.shaftOutputDirection.same  enable_faults=simscape.enum.onoff.off  efficiency_fault=0.05  fault_angles=pi / 12 rad  friction_model=sdl.enum.gear_efficiencies_load.off  T_noload=0.1 N*m  T_nom=5 N*m  efficiency_nom=0.8  efficiency=0.8  temperature_TLU=[280, 300, 320] K  load_TLU=[1, 5, 10] N*m  efficiency_TLU=[.95, .9, .85]  efficiency_TLU2=[.85, .8, .75; .95, .9, .85; .85, .8, .7]  w_thr=0.01 rad/s  pwr_thr=0.001 W  enable_backlash=false  hardstop_model=simscape.enum.hardstop.smooth  backlash_distance=1e-3 mm  r_base=0.1 m  transition=1e-4 mm  backlash_stiffness=1e6 N/m  backlash_damping=1e3 N*s/m  coeff_rest=0.7  v_tol=0.001 m/s  f_tol=0.001 N  mu_visc=[0, 0] N*m*s/rad  thermal_mass=50 J/K  temperature_specify=off  temperature_priority=High  temperature=300 K  temperature_nominal_specify=off  temperature_nominal_value=1  temperature_nominal_unit=K  x_backlash_specify=off  x_backlash_priority=None  x_backlash=0 mm  x_backlash_nominal_specify=off  x_backlash_nominal_value=1  x_backlash_nominal_unit=mm  f_hardstop_specify=off  f_hardstop_priority=None  f_hardstop=0 N  f_hardstop_nominal_specify=off  f_hardstop_nominal_value=1  f_hardstop_nominal_unit=N  v_backlash_specify=off  v_backlash_priority=None  v_backlash=0 m/s  v_backlash_nominal_specify=off  v_backlash_nominal_value=1  v_backlash_nominal_unit=m/s
  Solver Configuration : nesl_utility/Solver Configuration  PhysicalDomain=network_engine_domain  SubClassName=solver  LeftPortType=input  RightPortType=generic  Tones=[]  Harmonics=[]  SimulateNoise=off  Profile=off  UseLocalSampling=off  EnableSwitchedLinearOptims=on  FrequencyDomain=off  UseCCode=off  RelTol=0.001  AbsTol=0.001  MinStep=1e-09  ToWorkspace=off  RevertToSquareIcSolve=off  NumHomotopyIterations=100  PhasorMode=off  PhasorModeNumHarmonics=1  ConsistencySolver=NEWTON_XTOL_AFTER_FTOL  IndexReductionMethod=DerivativeReplacement  DoDC=off  ResidualTolerance=1e-09  ConsistencyTolSource=GLOBAL  ConsistencyAbsTol=0.001  ConsistencyRelTol=0.001  ConsistencyTolFactor=0.001  UseLocalSolver=off  LocalSolverChoice=NE_BACKWARD_EULER_ADVANCER  ResolveIndetEquations=on  FunctionEvalNumThread=1  LocalSolverSampleTime=0.001  DoFixedCost=off  MaxNonlinIter=3  MaxModeIter=2  ComputeImpulses=off  ImpulseIterations=2  LinearAlgebra=auto  LinearAlgebraNumThread=0  EquationFormulation=NE_TIME_EF  DelaysMemoryBudget=1024  AutomaticFiltering=on  FilteringTimeConstant=0.001  PartitionStorageMethod=AS_NEEDED  PartitionMemoryBudget=1024  PartitionMethod=ROBUST  MultibodyUseLocalSolver=off  MultibodyLocalSolverChoice=ODE1  MultibodyLocalSolverSampleTime=0.001
  Translational Multibody Interface : fl_lib/Mechanical/Multibody Interfaces/Translational Multibody Interface
  Voltage Source : ee_lib/Sources/Voltage Source  dc_voltage=48 %100 V  ac_voltage=0 V  ac_shift=0 rad  ac_frequency=60 Hz  noise_mode=ee.enum.sources.noise.Disabled  PSD=0 V^2/Hz  sample_time=1e-3 s  repeatability=ee.enum.sources.repeatability.NotRepeatable  user_seed=0  auto_seed=3890346746  i_specify=off  i_priority=None  i=0 A  i_nominal_specify=off  i_nominal_value=1  i_nominal_unit=A  v_specify=off  v_priority=None  v=0 V  v_nominal_specify=off  v_nominal_value=1  v_nominal_unit=V
  Wheel and Axle : fl_lib/Mechanical/Mechanisms/Wheel and Axle  R=0.071 m  or=1  t_specify=off  t_priority=None  t=0 N*m  t_nominal_specify=off  t_nominal_value=1  t_nominal_unit=N*m  f_specify=off  f_priority=None  f=0 N  f_nominal_specify=off  f_nominal_value=1  f_nominal_unit=N
  Motor Torque : PMIOPort  Side=Left
  Axis Velocity : PMIOPort  Port=2  Side=Left
  Actuator Force : PMIOPort  Port=3  Side=Right
  connections:
  Simple Gear/RConn1 -- Wheel and Axle/LConn1
  Inertia/LConn1 -- Rotational Damper/LConn1 -- Motor & Drive/LConn3 -- Simple Gear/LConn1
  Motor & Drive/LConn1 -- Voltage Source/LConn1
  Voltage Source/RConn1 -- Motor & Drive/RConn1 -- Electrical Reference/LConn1
  Mechanical Rotational Reference/LConn1 -- Motor & Drive/RConn3 -- Solver Configuration/RConn1 -- Rotational Damper/RConn1
  Motor & Drive/LConn2 -- Motor Torque/RConn1
  Translational Multibody Interface/RConn2 -- Wheel and Axle/RConn1
  Mechanical Translational Reference/LConn1 -- Translational Multibody Interface/LConn2
  Actuator Force/RConn1 -- Translational Multibody Interface/LConn1
  Axis Velocity/RConn1 -- Translational Multibody Interface/RConn1
